simulink model "NREL5MW_Baseline_fcnblock"  (Simulink 10.1)
settings: Solver=ode4  StartTime=0.0  StopTime=Parameter.Time.TMax  FixedStep=Parameter.Time.dt  RelTol=1e-3  EnableMultiTasking=on
undefined symbols (not defined in the file or in its folder): OutList, Parameter, strmatch, x2_t0
settings Model: Creator=Phoenix_Shao  LastModifiedBy=jveli
settings DataIOCC: MaxDataPoints=1000000  DSMLogging=off
settings OptimizationCC: ExpressionDepthLimit=2147483647  InitFltsAndDblsToZero=on  EfficientMapNaN2IntZero=off
settings DebuggingCC: SaveWithParameterizedLinksMsg=none  SignalResolutionControl=TryResolveAllWithWarning  SolverPrmCheckMsg=warning  MultiTaskDSMMsg=warning  MultiTaskCondExecSysMsg=none  FcnCallInpInsideContextMsg=warning  AllowSymbolicDim=off  StateNameClashWarn=warning
settings HardwareCC: TargetBitPerPointer=64  TargetBitPerSizeT=64  TargetBitPerPtrDiffT=64  TargetLongLongMode=on  TargetIntDivRoundTo=Zero  TargetEndianess=LittleEndian  TargetWordSize=64  TargetHWDeviceType=MATLAB Host  ProdEqTarget=off
settings SFSimCC: SimParseCustomCode=off
settings RTWCC: SystemTargetFile=accel.tlc  TemplateMakefile=accel_default_tmf  RTWVerbose=off
settings CodeAppCC: MaxIdLength=128
settings STFCustomTargetCC: MATLABClassNameForMDSCustomization=Simulink.SoftwareTarget.TargetSpecificTriggerConfigurationBase  SystemTargetFile=accel.tlc

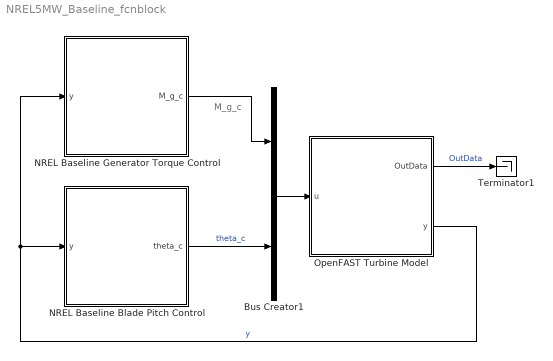
== system NREL5MW_Baseline_fcnblock ==
  note: M_g_c
  Bus Creator1 : BusCreator  Inputs=2
  NREL Baseline Blade Pitch Control : Subsystem
  NREL Baseline Generator Torque Control : Subsystem
  OpenFAST Turbine Model : Subsystem  AncestorBlock=Library/Models/FAST
  Terminator1 : Terminator
  wires:
  OpenFAST Turbine Model/2(y) -> NREL Baseline Generator Torque Control/1(y), NREL Baseline Blade Pitch Control/1(y)  "y"
  OpenFAST Turbine Model/1(OutData) -> Terminator1/1  "OutData"
  NREL Baseline Generator Torque Control/1(M_g_c) -> Bus Creator1/1
  Bus Creator1/1 -> OpenFAST Turbine Model/1(u)
  NREL Baseline Blade Pitch Control/1("theta_c ") -> Bus Creator1/2  "theta_c"

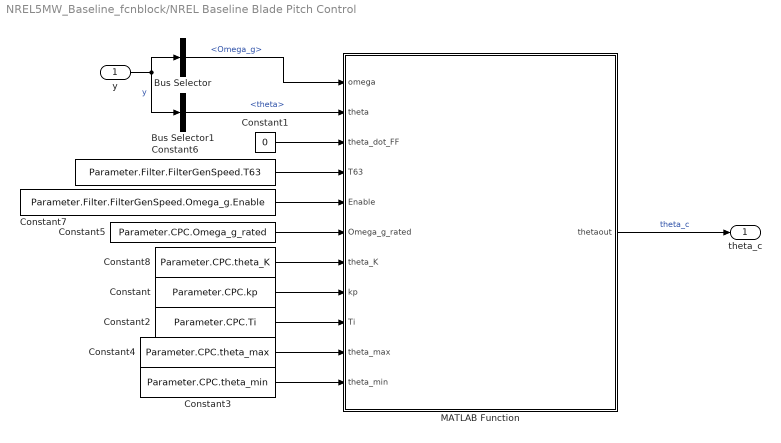
== system NREL5MW_Baseline_fcnblock/NREL Baseline Blade Pitch Control ==
  y : Inport
  Bus Selector : BusSelector  OutputSignals=Omega_g
  Bus Selector1 : BusSelector  OutputSignals=theta
  Constant : Constant  Value=Parameter.CPC.kp
  Constant1 : Constant  Value=0
  Constant2 : Constant  Value=Parameter.CPC.Ti
  Constant3 : Constant  Value=Parameter.CPC.theta_min
  Constant4 : Constant  Value=Parameter.CPC.theta_max
  Constant5 : Constant  Value=Parameter.CPC.Omega_g_rated
  Constant6 : Constant  Value=Parameter.Filter.FilterGenSpeed.T63
  Constant7 : Constant  Value=Parameter.Filter.FilterGenSpeed.Omega_g.Enable
  Constant8 : Constant  Value=Parameter.CPC.theta_K
  MATLAB Function : MATLAB Function  TreatAsAtomicUnit=on
  "theta_c " : Outport
  wires:
  y/1 -> Bus Selector/1, Bus Selector1/1  "y"
  Constant1/1 -> MATLAB Function/3(theta_dot_FF)
  MATLAB Function/1(thetaout) -> "theta_c "/1  "theta_c"
  Bus Selector/1 -> MATLAB Function/1(omega)  "<Omega_g>"
  Bus Selector1/1 -> MATLAB Function/2(theta)  "<theta>"
  Constant6/1 -> MATLAB Function/4(T63)
  Constant7/1 -> MATLAB Function/5(Enable)
  Constant3/1 -> MATLAB Function/11(theta_min)
  Constant4/1 -> MATLAB Function/10(theta_max)
  Constant5/1 -> MATLAB Function/6(Omega_g_rated)
  Constant/1 -> MATLAB Function/8(kp)
  Constant8/1 -> MATLAB Function/7(theta_K)
  Constant2/1 -> MATLAB Function/9(Ti)

== system NREL5MW_Baseline_fcnblock/NREL Baseline Generator Torque Control ==
  y : Inport
  Bus Selector : BusSelector  OutputSignals=Omega_g
  Bus Selector1 : BusSelector  OutputSignals=theta
  FilterGenSpeed.Omega_g : Subsystem
  NREL 5MW BaselineTorque Controller : Subsystem
  M_g_c : Outport
  wires:
  FilterGenSpeed.Omega_g/1(y) -> NREL 5MW BaselineTorque Controller/1(Omega_g [rad/s])
  Bus Selector1/1 -> NREL 5MW BaselineTorque Controller/2(theta [rad])  "<theta>"
  Bus Selector/1 -> FilterGenSpeed.Omega_g/1(u)  "<Omega_g>"
  y/1 -> Bus Selector/1, Bus Selector1/1  "y"
  NREL 5MW BaselineTorque Controller/1(M_g [Nm]) -> M_g_c/1  "M_g_c"

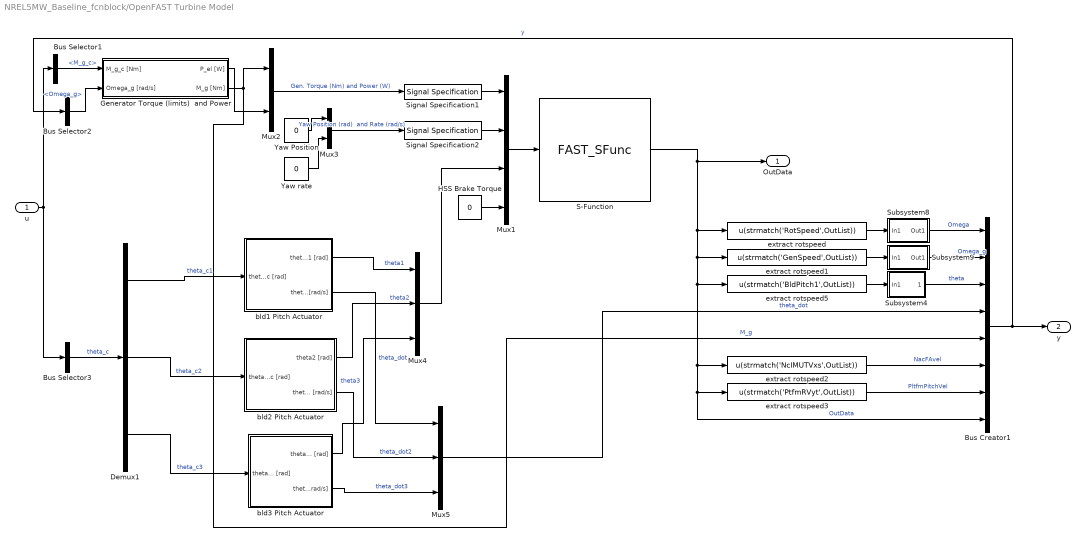
== system NREL5MW_Baseline_fcnblock/OpenFAST Turbine Model ==
  u : Inport
  Bus Creator1 : BusCreator  Inputs=8
  Bus Selector1 : BusSelector  OutputSignals=M_g_c
  Bus Selector2 : BusSelector  OutputSignals=Omega_g
  Bus Selector3 : BusSelector  OutputSignals=theta_c  OutputAsBus=on
  Demux1 : Demux  Outputs=3
  Generator Torque (limits)  and Power : Subsystem  AncestorBlock=Library/Models/Generator
  HSS Brake Torque : Constant  Value=0
  Mux1 : Mux
  Mux2 : Mux  Inputs=2
  Mux3 : Mux  Inputs=2
  Mux4 : Mux  Inputs=3
  Mux5 : Mux  Inputs=3
  S-Function : S-Function  FunctionName=FAST_SFunc  Parameters=Parameter.FASTfile, Parameter.Time.TMax, 0  SFunctionDeploymentMode=off  EnableBusSupport=off
  Signal Specification1 : SignalSpecification  OutDataTypeStr=double  Dimensions=2
  Signal Specification2 : SignalSpecification  OutDataTypeStr=double  Dimensions=2
  Subsystem4 : Subsystem
      mask Display: disp('deg2rad')
  Subsystem8 : Subsystem
      mask Display: disp('rpm2rad/s')
  Subsystem9 : Subsystem
      mask Display: disp('rpm2rad/s')
  Yaw Position : Constant  Value=0
  Yaw rate : Constant  Value=0
  bld1 Pitch Actuator : Subsystem  AncestorBlock=Library/Models/Pitch Actuator
  bld2 Pitch Actuator : Subsystem  AncestorBlock=Library/Models/Pitch Actuator
  bld3 Pitch Actuator : Subsystem  AncestorBlock=Library/Models/Pitch Actuator
  extract rotspeed : Fcn  Expr=u(strmatch('RotSpeed',OutList))
  extract rotspeed1 : Fcn  Expr=u(strmatch('GenSpeed',OutList))
  extract rotspeed2 : Fcn  Expr=u(strmatch('NcIMUTVxs',OutList))
  extract rotspeed3 : Fcn  Expr=u(strmatch('PtfmRVyt',OutList))
  extract rotspeed5 : Fcn  Expr=u(strmatch('BldPitch1',OutList))
  OutData : Outport
  y : Outport  Port=2
  wires:
  Subsystem9/1(Out1) -> Bus Creator1/2  "Omega_g"
  Subsystem8/1(Out1) -> Bus Creator1/1  "Omega"
  extract rotspeed5/1 -> Subsystem4/1(In1)
  Bus Creator1/1 -> y/1, Bus Selector2/1  "y"
  extract rotspeed1/1 -> Subsystem9/1(In1)
  extract rotspeed/1 -> Subsystem8/1(In1)
  Subsystem4/1(Out1) -> Bus Creator1/3  "theta"
  Bus Selector1/1 -> Generator Torque (limits)  and Power/1(M_g_c [Nm])  "<M_g_c>"
  Mux4/1 -> Mux1/3
  u/1 -> Bus Selector3/1, Bus Selector1/1
  Mux2/1 -> Signal Specification1/1  "Gen. Torque (Nm) and Power (W)"
  S-Function/1 -> Bus Creator1/8, extract rotspeed3/1, extract rotspeed2/1, extract rotspeed5/1, extract rotspeed1/1, extract rotspeed/1, OutData/1  "OutData"
  Mux1/1 -> S-Function/1
  Mux3/1 -> Signal Specification2/1  "Yaw Position (rad)  and Rate (rad/s)"
  Signal Specification1/1 -> Mux1/1
  Signal Specification2/1 -> Mux1/2
  Yaw Position/1 -> Mux3/1
  Yaw rate/1 -> Mux3/2
  Bus Selector2/1 -> Generator Torque (limits)  and Power/2(Omega_g [rad/s])  "<Omega_g>"
  Generator Torque (limits)  and Power/1(P_el [W]) -> Mux2/2
  Generator Torque (limits)  and Power/2(M_g [Nm]) -> Mux2/1, Bus Creator1/5  "M_g"
  HSS Brake Torque/1 -> Mux1/4
  extract rotspeed2/1 -> Bus Creator1/6  "NacFAvel"
  extract rotspeed3/1 -> Bus Creator1/7  "PltfmPitchVel"
  bld1 Pitch Actuator/1(theta1 [rad]) -> Mux4/1  "theta1"
  bld2 Pitch Actuator/1(theta2 [rad]) -> Mux4/2  "theta2"
  bld1 Pitch Actuator/2(theta_dot1 [rad/s]) -> Mux5/1  "theta_dot"
  bld2 Pitch Actuator/2(theta_dot2 [rad/s]) -> Mux5/2  "theta_dot2"
  bld3 Pitch Actuator/2(theta_dot3 [rad/s]) -> Mux5/3  "theta_dot3"
  bld3 Pitch Actuator/1(theta3 [rad]) -> Mux4/3  "theta3"
  Bus Selector3/1 -> Demux1/1  "theta_c"
  Demux1/1 -> bld1 Pitch Actuator/1(theta_c [rad])  "theta_c1"
  Demux1/2 -> bld2 Pitch Actuator/1(theta_c [rad])  "theta_c2"
  Demux1/3 -> bld3 Pitch Actuator/1(theta_c [rad])  "theta_c3"
  Mux5/1 -> Bus Creator1/4  "theta_dot"

== system NREL5MW_Baseline_fcnblock/NREL Baseline Generator Torque Control/FilterGenSpeed.Omega_g ==
  u : Inport
  Constant1 : Constant  Value=Parameter.Filter.FilterGenSpeed.T63
  Constant3 : Constant  Value=Parameter.Filter.FilterGenSpeed.Omega_g.Enable
  LowPassOrder1 : Subsystem
  y : Outport
  wires:
  LowPassOrder1/1(y) -> y/1
  u/1 -> LowPassOrder1/2(u), LowPassOrder1/1(u0)
  Constant3/1 -> LowPassOrder1/4(Enable)
  Constant1/1 -> LowPassOrder1/3(T)

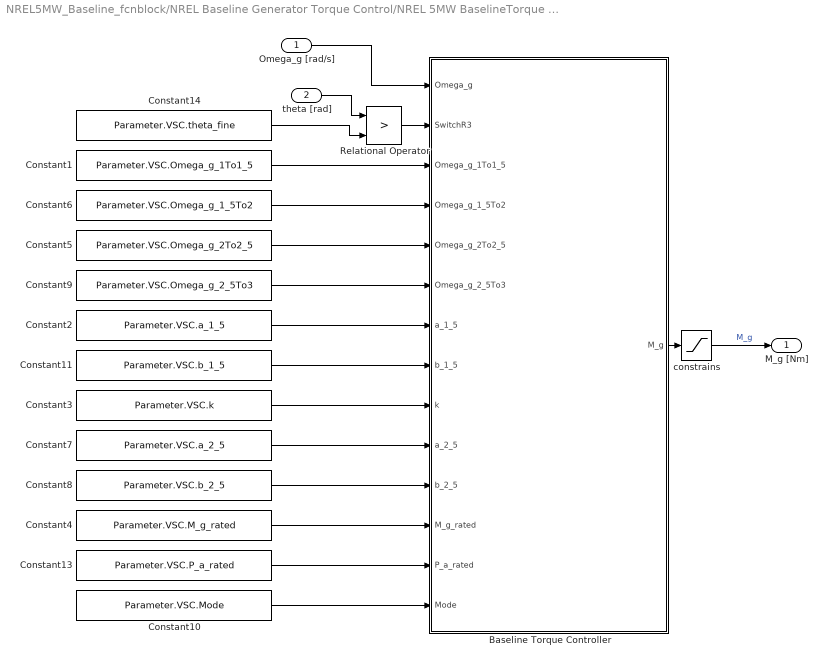
== system NREL5MW_Baseline_fcnblock/NREL Baseline Generator Torque Control/NREL 5MW BaselineTorque Controller ==
  Omega_g [rad/s] : Inport
  theta [rad] : Inport  Port=2
  Baseline Torque Controller : MATLAB Function  TreatAsAtomicUnit=on
  Constant1 : Constant  Value=Parameter.VSC.Omega_g_1To1_5
  Constant10 : Constant  Value=Parameter.VSC.Mode
  Constant11 : Constant  Value=Parameter.VSC.b_1_5
  Constant13 : Constant  Value=Parameter.VSC.P_a_rated
  Constant14 : Constant  Value=Parameter.VSC.theta_fine
  Constant2 : Constant  Value=Parameter.VSC.a_1_5
  Constant3 : Constant  Value=Parameter.VSC.k
  Constant4 : Constant  Value=Parameter.VSC.M_g_rated
  Constant5 : Constant  Value=Parameter.VSC.Omega_g_2To2_5
  Constant6 : Constant  Value=Parameter.VSC.Omega_g_1_5To2
  Constant7 : Constant  Value=Parameter.VSC.a_2_5
  Constant8 : Constant  Value=Parameter.VSC.b_2_5
  Constant9 : Constant  Value=Parameter.VSC.Omega_g_2_5To3
  Relational Operator : RelationalOperator  Operator=>  OutDataTypeStr=boolean  RndMeth=Nearest
  constrains : Saturate  UpperLimit=Parameter.VSC.M_g_max  LowerLimit=Parameter.VSC.M_g_min
  M_g [Nm] : Outport
  wires:
  Constant13/1 -> Baseline Torque Controller/13(P_a_rated)
  Constant11/1 -> Baseline Torque Controller/8(b_1_5)
  Constant2/1 -> Baseline Torque Controller/7(a_1_5)
  Constant10/1 -> Baseline Torque Controller/14(Mode)
  Constant3/1 -> Baseline Torque Controller/9(k)
  Constant7/1 -> Baseline Torque Controller/10(a_2_5)
  Constant8/1 -> Baseline Torque Controller/11(b_2_5)
  Constant4/1 -> Baseline Torque Controller/12(M_g_rated)
  Constant9/1 -> Baseline Torque Controller/6(Omega_g_2_5To3)
  Constant6/1 -> Baseline Torque Controller/4(Omega_g_1_5To2)
  Constant5/1 -> Baseline Torque Controller/5(Omega_g_2To2_5)
  Constant1/1 -> Baseline Torque Controller/3(Omega_g_1To1_5)
  constrains/1 -> M_g [Nm]/1  "M_g"
  Omega_g [rad/s]/1 -> Baseline Torque Controller/1(Omega_g)
  Baseline Torque Controller/1(M_g) -> constrains/1
  Constant14/1 -> Relational Operator/2
  theta [rad]/1 -> Relational Operator/1
  Relational Operator/1 -> Baseline Torque Controller/2(SwitchR3)

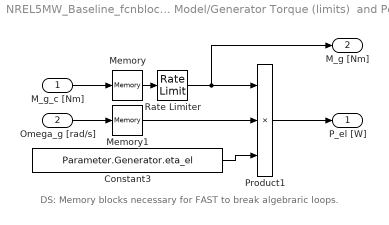
== system NREL5MW_Baseline_fcnblock/OpenFAST Turbine Model/Generator Torque (limits)  and Power ==
  note: DS: Memory blocks necessary for FAST to break algebraric loops.
  M_g_c [Nm] : Inport
  Omega_g [rad/s] : Inport  Port=2
  Constant3 : Constant  Value=Parameter.Generator.eta_el
  Memory : Memory  InitialCondition=Parameter.IC.M_g
  Memory1 : Memory  InitialCondition=Parameter.IC.Omega/Parameter.Turbine.i
  Product1 : Product  Inputs=***  RndMeth=Zero
  Rate Limiter : RateLimiter  RisingSlewLimit=Parameter.Generator.M_g_dot_max  FallingSlewLimit=-Parameter.Generator.M_g_dot_max  SampleTimeMode=inherited  InitialCondition=Parameter.IC.M_g
  P_el [W] : Outport
  M_g [Nm] : Outport  Port=2
  wires:
  Memory1/1 -> Product1/2
  Memory/1 -> Rate Limiter/1
  Omega_g [rad/s]/1 -> Memory1/1
  Rate Limiter/1 -> M_g [Nm]/1, Product1/1
  Constant3/1 -> Product1/3
  M_g_c [Nm]/1 -> Memory/1
  Product1/1 -> P_el [W]/1

== system NREL5MW_Baseline_fcnblock/OpenFAST Turbine Model/Subsystem4 ==
  In1 : Inport
  deg in rad : Gain  Gain=2*pi/360  SaturateOnIntegerOverflow=on  OutDataTypeStr=Inherit: Same as input  ParamDataTypeStr=Inherit: Same as input
  Out1 : Outport
  wires:
  In1/1 -> deg in rad/1
  deg in rad/1 -> Out1/1

== system NREL5MW_Baseline_fcnblock/OpenFAST Turbine Model/Subsystem8 ==
  In1 : Inport
  rpm in rad/s : Gain  Gain=2*pi/60  SaturateOnIntegerOverflow=on  OutDataTypeStr=Inherit: Same as input  ParamDataTypeStr=Inherit: Same as input
  Out1 : Outport
  wires:
  rpm in rad/s/1 -> Out1/1
  In1/1 -> rpm in rad/s/1

== system NREL5MW_Baseline_fcnblock/OpenFAST Turbine Model/Subsystem9 ==
  In1 : Inport
  rpm in rad/s : Gain  Gain=2*pi/60  SaturateOnIntegerOverflow=on  OutDataTypeStr=Inherit: Same as input  ParamDataTypeStr=Inherit: Same as input
  Out1 : Outport
  wires:
  In1/1 -> rpm in rad/s/1
  rpm in rad/s/1 -> Out1/1

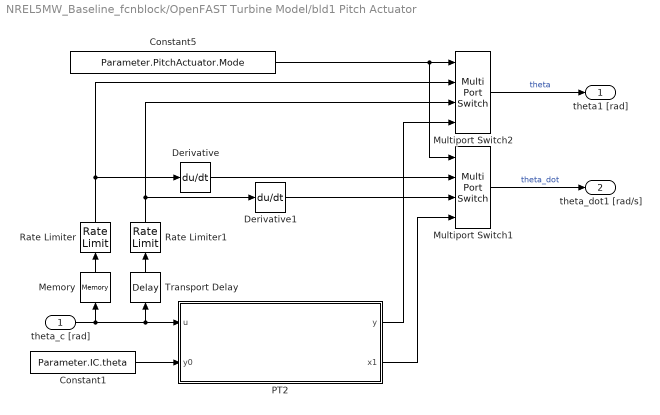
== system NREL5MW_Baseline_fcnblock/OpenFAST Turbine Model/bld1 Pitch Actuator ==
  theta_c [rad] : Inport
  Constant1 : Constant  Value=Parameter.IC.theta
  Constant5 : Constant  Value=Parameter.PitchActuator.Mode
  Derivative : Derivative
  Derivative1 : Derivative
  Memory : Memory  InitialCondition=Parameter.IC.theta
  Multiport Switch1 : MultiPortSwitch  DataPortOrder=Specify indices  DataPortIndices={0,1,2}
  Multiport Switch2 : MultiPortSwitch  DataPortOrder=Specify indices  DataPortIndices={0,1,2}
  PT2 : Subsystem  mask{omega=Parameter.PitchActuator.omega, xi=Parameter.PitchActuator.xi, x1_max=Parameter.PitchActuator.theta_dot_max, x1_min=-Parameter.PitchActuator.theta_dot_max, x2_max=Parameter.PitchActuator.theta_max, x2_min=Parameter.PitchActuator.theta_min}
      mask prompts: omega "undamped natural frequency [rad/s]"; xi "damping factor [-]"; x1_max "Upper bound x1"; x1_min "Lower bound x1"; x2_max "Upper bound x2"; x2_min "Lower bound x2"
      mask Display:
      | disp(['omega = ',num2str(omega),'\n'...
      |     ,'xi = ',num2str(xi)])
      | port_label('output',1,'y')
      | port_label('output',2,'x1')
      | port_label('input',2,'y0')
      | port_label('input',1,'u')
  Rate Limiter : RateLimiter  RisingSlewLimit=Parameter.PitchActuator.theta_dot_max  FallingSlewLimit=-Parameter.PitchActuator.theta_dot_max  SampleTimeMode=inherited  InitialCondition=Parameter.IC.theta
  Rate Limiter1 : RateLimiter  RisingSlewLimit=Parameter.PitchActuator.theta_dot_max  FallingSlewLimit=-Parameter.PitchActuator.theta_dot_max  SampleTimeMode=inherited  InitialCondition=Parameter.IC.theta
  Transport Delay : TransportDelay  DelayTime=Parameter.PitchActuator.Delay  InitialOutput=Parameter.IC.theta
  theta1 [rad] : Outport
  theta_dot1 [rad/s] : Outport  Port=2
  wires:
  Constant1/1 -> PT2/2(y0)
  Rate Limiter1/1 -> Multiport Switch2/3, Derivative1/1
  Transport Delay/1 -> Rate Limiter1/1
  Derivative1/1 -> Multiport Switch1/3
  PT2/2(x1) -> Multiport Switch1/4
  theta_c [rad]/1 -> PT2/1(u), Transport Delay/1, Memory/1
  Constant5/1 -> Multiport Switch2/1, Multiport Switch1/1
  Multiport Switch2/1 -> theta1 [rad]/1  "theta"
  Derivative/1 -> Multiport Switch1/2
  Multiport Switch1/1 -> theta_dot1 [rad/s]/1  "theta_dot"
  Rate Limiter/1 -> Derivative/1, Multiport Switch2/2
  Memory/1 -> Rate Limiter/1
  PT2/1(y) -> Multiport Switch2/4

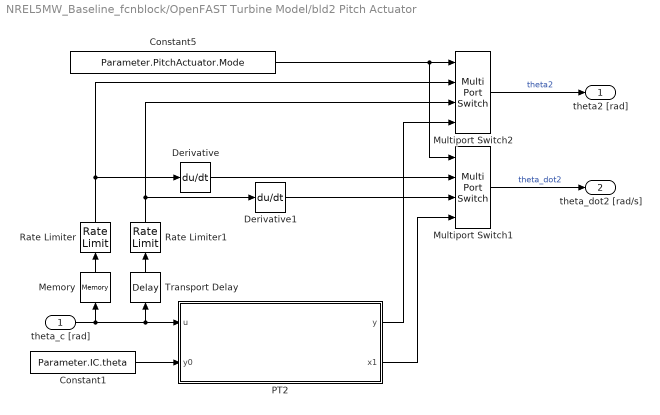
== system NREL5MW_Baseline_fcnblock/OpenFAST Turbine Model/bld2 Pitch Actuator ==
  theta_c [rad] : Inport
  Constant1 : Constant  Value=Parameter.IC.theta
  Constant5 : Constant  Value=Parameter.PitchActuator.Mode
  Derivative : Derivative
  Derivative1 : Derivative
  Memory : Memory  InitialCondition=Parameter.IC.theta
  Multiport Switch1 : MultiPortSwitch  DataPortOrder=Specify indices  DataPortIndices={0,1,2}
  Multiport Switch2 : MultiPortSwitch  DataPortOrder=Specify indices  DataPortIndices={0,1,2}
  PT2 : Subsystem  mask{omega=Parameter.PitchActuator.omega, xi=Parameter.PitchActuator.xi, x1_max=Parameter.PitchActuator.theta_dot_max, x1_min=-Parameter.PitchActuator.theta_dot_max, x2_max=Parameter.PitchActuator.theta_max, x2_min=Parameter.PitchActuator.theta_min}
      mask prompts: omega "undamped natural frequency [rad/s]"; xi "damping factor [-]"; x1_max "Upper bound x1"; x1_min "Lower bound x1"; x2_max "Upper bound x2"; x2_min "Lower bound x2"
      mask Display:
      | disp(['omega = ',num2str(omega),'\n'...
      |     ,'xi = ',num2str(xi)])
      | port_label('output',1,'y')
      | port_label('output',2,'x1')
      | port_label('input',2,'y0')
      | port_label('input',1,'u')
  Rate Limiter : RateLimiter  RisingSlewLimit=Parameter.PitchActuator.theta_dot_max  FallingSlewLimit=-Parameter.PitchActuator.theta_dot_max  SampleTimeMode=inherited  InitialCondition=Parameter.IC.theta
  Rate Limiter1 : RateLimiter  RisingSlewLimit=Parameter.PitchActuator.theta_dot_max  FallingSlewLimit=-Parameter.PitchActuator.theta_dot_max  SampleTimeMode=inherited  InitialCondition=Parameter.IC.theta
  Transport Delay : TransportDelay  DelayTime=Parameter.PitchActuator.Delay  InitialOutput=Parameter.IC.theta
  theta2 [rad] : Outport
  theta_dot2 [rad/s] : Outport  Port=2
  wires:
  Constant1/1 -> PT2/2(y0)
  Rate Limiter1/1 -> Multiport Switch2/3, Derivative1/1
  Transport Delay/1 -> Rate Limiter1/1
  Derivative1/1 -> Multiport Switch1/3
  PT2/2(x1) -> Multiport Switch1/4
  theta_c [rad]/1 -> PT2/1(u), Transport Delay/1, Memory/1
  Constant5/1 -> Multiport Switch2/1, Multiport Switch1/1
  Multiport Switch2/1 -> theta2 [rad]/1  "theta2"
  Derivative/1 -> Multiport Switch1/2
  Multiport Switch1/1 -> theta_dot2 [rad/s]/1  "theta_dot2"
  Rate Limiter/1 -> Derivative/1, Multiport Switch2/2
  Memory/1 -> Rate Limiter/1
  PT2/1(y) -> Multiport Switch2/4

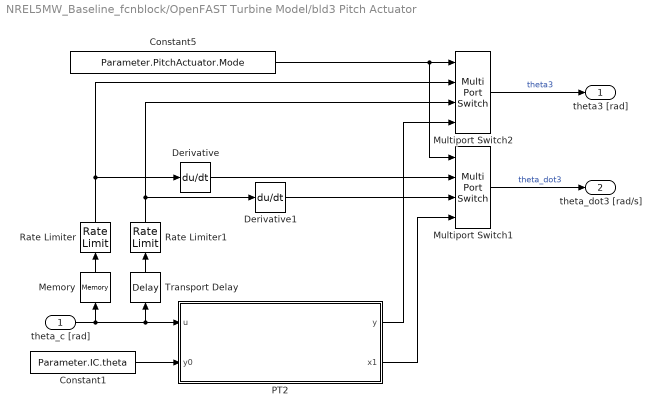
== system NREL5MW_Baseline_fcnblock/OpenFAST Turbine Model/bld3 Pitch Actuator ==
  theta_c [rad] : Inport
  Constant1 : Constant  Value=Parameter.IC.theta
  Constant5 : Constant  Value=Parameter.PitchActuator.Mode
  Derivative : Derivative
  Derivative1 : Derivative
  Memory : Memory  InitialCondition=Parameter.IC.theta
  Multiport Switch1 : MultiPortSwitch  DataPortOrder=Specify indices  DataPortIndices={0,1,2}
  Multiport Switch2 : MultiPortSwitch  DataPortOrder=Specify indices  DataPortIndices={0,1,2}
  PT2 : Subsystem  mask{omega=Parameter.PitchActuator.omega, xi=Parameter.PitchActuator.xi, x1_max=Parameter.PitchActuator.theta_dot_max, x1_min=-Parameter.PitchActuator.theta_dot_max, x2_max=Parameter.PitchActuator.theta_max, x2_min=Parameter.PitchActuator.theta_min}
      mask prompts: omega "undamped natural frequency [rad/s]"; xi "damping factor [-]"; x1_max "Upper bound x1"; x1_min "Lower bound x1"; x2_max "Upper bound x2"; x2_min "Lower bound x2"
      mask Display:
      | disp(['omega = ',num2str(omega),'\n'...
      |     ,'xi = ',num2str(xi)])
      | port_label('output',1,'y')
      | port_label('output',2,'x1')
      | port_label('input',2,'y0')
      | port_label('input',1,'u')
  Rate Limiter : RateLimiter  RisingSlewLimit=Parameter.PitchActuator.theta_dot_max  FallingSlewLimit=-Parameter.PitchActuator.theta_dot_max  SampleTimeMode=inherited  InitialCondition=Parameter.IC.theta
  Rate Limiter1 : RateLimiter  RisingSlewLimit=Parameter.PitchActuator.theta_dot_max  FallingSlewLimit=-Parameter.PitchActuator.theta_dot_max  SampleTimeMode=inherited  InitialCondition=Parameter.IC.theta
  Transport Delay : TransportDelay  DelayTime=Parameter.PitchActuator.Delay  InitialOutput=Parameter.IC.theta
  theta3 [rad] : Outport
  theta_dot3 [rad/s] : Outport  Port=2
  wires:
  Constant1/1 -> PT2/2(y0)
  Rate Limiter1/1 -> Multiport Switch2/3, Derivative1/1
  Transport Delay/1 -> Rate Limiter1/1
  Derivative1/1 -> Multiport Switch1/3
  PT2/2(x1) -> Multiport Switch1/4
  theta_c [rad]/1 -> PT2/1(u), Transport Delay/1, Memory/1
  Constant5/1 -> Multiport Switch2/1, Multiport Switch1/1
  Multiport Switch2/1 -> theta3 [rad]/1  "theta3"
  Derivative/1 -> Multiport Switch1/2
  Multiport Switch1/1 -> theta_dot3 [rad/s]/1  "theta_dot3"
  Rate Limiter/1 -> Derivative/1, Multiport Switch2/2
  Memory/1 -> Rate Limiter/1
  PT2/1(y) -> Multiport Switch2/4

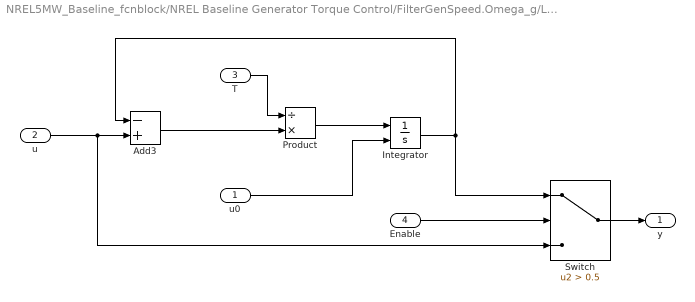
== system NREL5MW_Baseline_fcnblock/NREL Baseline Generator Torque Control/FilterGenSpeed.Omega_g/LowPassOrder1 ==
  u0 : Inport
  u : Inport  Port=2
  T : Inport  Port=3
  Enable : Inport  Port=4
  Add3 : Sum  Inputs=-+
  Integrator : Integrator  InitialConditionSource=external
  Product : Product  Inputs=/*  RndMeth=Zero
  Switch : Switch  Criteria=u2 > Threshold  Threshold=0.5
  y : Outport
  wires:
  u0/1 -> Integrator/2
  Switch/1 -> y/1
  Enable/1 -> Switch/2
  u/1 -> Add3/2, Switch/3
  T/1 -> Product/1
  Integrator/1 -> Add3/1, Switch/1
  Product/1 -> Integrator/1
  Add3/1 -> Product/2

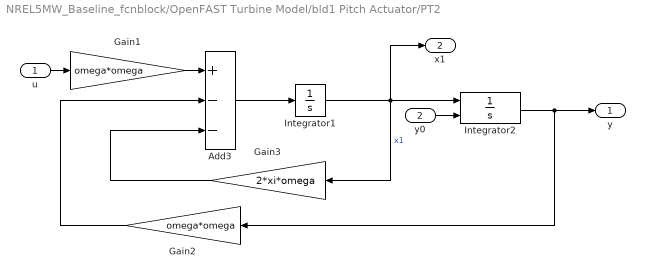
== system NREL5MW_Baseline_fcnblock/OpenFAST Turbine Model/bld1 Pitch Actuator/PT2 ==
  u : Inport
  y0 : Inport  Port=2
  Add3 : Sum  Inputs=+--
  Gain1 : Gain  Gain=omega*omega  SaturateOnIntegerOverflow=on  OutDataTypeStr=Inherit: Same as input  ParamDataTypeStr=Inherit: Same as input
  Gain2 : Gain  Gain=omega*omega  SaturateOnIntegerOverflow=on  OutDataTypeStr=Inherit: Same as input  ParamDataTypeStr=Inherit: Same as input
  Gain3 : Gain  Gain=2*xi*omega  SaturateOnIntegerOverflow=on  OutDataTypeStr=Inherit: Same as input  ParamDataTypeStr=Inherit: Same as input
  Integrator1 : Integrator  LimitOutput=on  UpperSaturationLimit=x1_max  LowerSaturationLimit=x1_min
  Integrator2 : Integrator  InitialConditionSource=external  InitialCondition=x2_t0  LimitOutput=on  UpperSaturationLimit=x2_max  LowerSaturationLimit=x2_min
  y : Outport
  x1 : Outport  Port=2
  wires:
  Integrator2/1 -> y/1, Gain2/1
  y0/1 -> Integrator2/2
  Integrator1/1 -> Integrator2/1, Gain3/1, x1/1  "x1"
  Gain2/1 -> Add3/2
  Gain1/1 -> Add3/1
  Add3/1 -> Integrator1/1
  u/1 -> Gain1/1
  Gain3/1 -> Add3/3

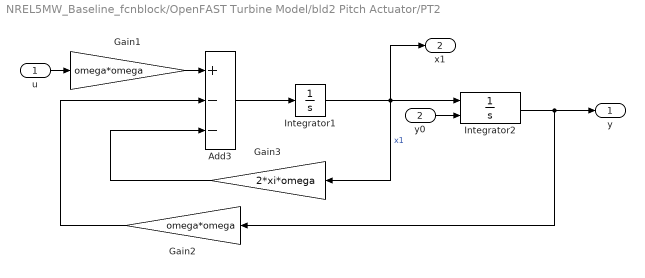
== system NREL5MW_Baseline_fcnblock/OpenFAST Turbine Model/bld2 Pitch Actuator/PT2 ==
  u : Inport
  y0 : Inport  Port=2
  Add3 : Sum  Inputs=+--
  Gain1 : Gain  Gain=omega*omega  SaturateOnIntegerOverflow=on  OutDataTypeStr=Inherit: Same as input  ParamDataTypeStr=Inherit: Same as input
  Gain2 : Gain  Gain=omega*omega  SaturateOnIntegerOverflow=on  OutDataTypeStr=Inherit: Same as input  ParamDataTypeStr=Inherit: Same as input
  Gain3 : Gain  Gain=2*xi*omega  SaturateOnIntegerOverflow=on  OutDataTypeStr=Inherit: Same as input  ParamDataTypeStr=Inherit: Same as input
  Integrator1 : Integrator  LimitOutput=on  UpperSaturationLimit=x1_max  LowerSaturationLimit=x1_min
  Integrator2 : Integrator  InitialConditionSource=external  InitialCondition=x2_t0  LimitOutput=on  UpperSaturationLimit=x2_max  LowerSaturationLimit=x2_min
  y : Outport
  x1 : Outport  Port=2
  wires:
  Integrator2/1 -> y/1, Gain2/1
  y0/1 -> Integrator2/2
  Integrator1/1 -> Integrator2/1, Gain3/1, x1/1  "x1"
  Gain2/1 -> Add3/2
  Gain1/1 -> Add3/1
  Add3/1 -> Integrator1/1
  u/1 -> Gain1/1
  Gain3/1 -> Add3/3

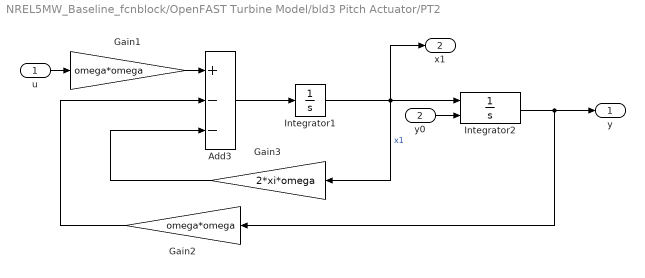
== system NREL5MW_Baseline_fcnblock/OpenFAST Turbine Model/bld3 Pitch Actuator/PT2 ==
  u : Inport
  y0 : Inport  Port=2
  Add3 : Sum  Inputs=+--
  Gain1 : Gain  Gain=omega*omega  SaturateOnIntegerOverflow=on  OutDataTypeStr=Inherit: Same as input  ParamDataTypeStr=Inherit: Same as input
  Gain2 : Gain  Gain=omega*omega  SaturateOnIntegerOverflow=on  OutDataTypeStr=Inherit: Same as input  ParamDataTypeStr=Inherit: Same as input
  Gain3 : Gain  Gain=2*xi*omega  SaturateOnIntegerOverflow=on  OutDataTypeStr=Inherit: Same as input  ParamDataTypeStr=Inherit: Same as input
  Integrator1 : Integrator  LimitOutput=on  UpperSaturationLimit=x1_max  LowerSaturationLimit=x1_min
  Integrator2 : Integrator  InitialConditionSource=external  InitialCondition=x2_t0  LimitOutput=on  UpperSaturationLimit=x2_max  LowerSaturationLimit=x2_min
  y : Outport
  x1 : Outport  Port=2
  wires:
  Integrator2/1 -> y/1, Gain2/1
  y0/1 -> Integrator2/2
  Integrator1/1 -> Integrator2/1, Gain3/1, x1/1  "x1"
  Gain2/1 -> Add3/2
  Gain1/1 -> Add3/1
  Add3/1 -> Integrator1/1
  u/1 -> Gain1/1
  Gain3/1 -> Add3/3

== matlab function NREL Baseline Generator Torque Control/NREL 5MW BaselineTorque Controller/Baseline Torque Controller ==
  settings: fimath=|
      | fimath(...
      | 'RoundMode', 'floor',...
      | 'OverflowMode', 'wrap',...
      | 'ProductMode', 'KeepLSB', 'ProductWordLength', 32,...
      | 'SumMode', 'KeepLSB', 'SumWordLength', 32,...
      | 'CastBeforeSum', false)
  data: Omega_g input double; SwitchR3 input double; Omega_g_1To1_5 input double; Omega_g_1_5To2 input double; Omega_g_2To2_5 input double; Omega_g_2_5To3 input double; a_1_5 input double; b_1_5 input double; k input double; a_2_5 input double; b_2_5 input double; M_g output double; M_g_rated input double; P_a_rated input double; Mode input double
function M_g = BaselineVSControl(Omega_g,SwitchR3,...  	% signals
    Omega_g_1To1_5,Omega_g_1_5To2,...
    Omega_g_2To2_5,Omega_g_2_5To3,...                   % region limits
    a_1_5,b_1_5,...                                    	% Region 1.5 parameters
    k,...                                             	% Region   2 parameters
    a_2_5,b_2_5,...                                    	% Region 2.5 parameters
    M_g_rated,P_a_rated,Mode)                        	% Region   3 parameters

if  Mode == 1                                         	% Power constant
    M_g_3 = P_a_rated/Omega_g;
else                                                    % Torque constant
    M_g_3 = M_g_rated;
end

if      Omega_g_2_5To3  <   Omega_g                     % Region 3
    M_g     = M_g_3;

elseif  Omega_g_2To2_5  <   Omega_g                     % Region 2.5
    M_g_2_5 = a_2_5 * Omega_g + b_2_5;
    M_g     = SwitchR3*M_g_3+(1-SwitchR3)*M_g_2_5;

elseif  Omega_g_1_5To2  <   Omega_g                     % Region 2
    M_g_2   = k * Omega_g^2;
    M_g     = SwitchR3*M_g_3+(1-SwitchR3)*M_g_2;  
    
elseif  Omega_g_1To1_5  <   Omega_g                     % Region 1.5
    M_g = a_1_5 * Omega_g + b_1_5;

else                                                    % Region 1 
    M_g = 0;    
end

== matlab function NREL Baseline Blade Pitch Control/MATLAB Function ==
  data: omega input double; thetaout output double; theta input double; theta_dot_FF input double; T63 input double; Enable input double; Omega_g_rated input double; theta_K input double; kp input double; Ti input double; theta_max input double; theta_min input double
function thetaout = Baseline_fcnblock(omega,theta,theta_dot_FF,T63,Enable,Omega_g_rated,theta_K,kp,Ti,theta_max,theta_min)

%% FilterGenSpeet Block (uses state X1)
%Define persistant Variable
persistent X1
if isempty(X1)
    X1 = 1;
    X0 = omega;
end

X1_dot = 1/T63*(omega - X0 * X1); %cheese it since we cannot define X1 in terms of an input
 
omega_filter = X0 * X1;

X1 = X1 + X1_dot;
X0 = 1;             %cancel out initial condition                   

%Calculate X1_dot
if Enable > .5
else
   omega_filter = omega; 
end

%% CPC controler Block (Uses State X2)
persistent X2
if isempty(X2)
    X2 = 1;
    X0_2 = theta;
end

%error signal
Error = (omega_filter - Omega_g_rated)/(1 + theta/theta_K);

X2_dot = 1/Ti*(fminmax(X0_2 * X2 + Error * kp,theta_max,theta_min) - X0_2 * X2) + theta_dot_FF; 

%output
thetaout = fminmax(X0_2 * X2 + Error * kp,theta_max,theta_min);
thetaout = [thetaout ; thetaout ; thetaout];   %all pitches the same

%next step in SS
X2 = X21 + X2_dot;
X0_2 = 1;                  %cancel out initial condition after first pass through function 


end

function y = fminmax(u,theta_max,theta_min)
y = u;
if u > theta_max
    y = theta_max;
end
if u < theta_min
    y = theta_min;
end    


end
